simulink model "sampleModel653"  (R2023a)
settings: Solver=VariableStepAuto  StartTime=0.0  StopTime=10.0  RelTol=1e-3
undefined symbols (not defined in the file): DiscIntNeverNeededParam, magnitude, Newton, Raphson
libraries: simulink x238, slpidlib x68
(part 5 of 11)

== system sampleModel653/cfblk133/cfblk4 ==
  cfblk1 : Inport
  cfblk10 : Gain  Gain=[-367085612.698275]
  cfblk11 : Delay  SampleTime=1
  cfblk3 : DiscreteTransferFcn  SampleTime=1
  cfblk4 : Delay  DelayLengthSource=Input port  SampleTime=1
      settings: InputPortMap=u0,p1
  cfblk5 : simulink/Discrete/Transfer Fcn First Order  PoleZ=0.95  ICPrevOutput=0.0  DoSatur=off
  cfblk6 : Polyval  Coefs=[ +2.081618890e-019, -1.441693666e-014, +4.719686976e-010, -8.536869453e-006, +1.621573104e-001, -8.087801117e+001 ]
  cfblk7 : Product  Inputs=*
  cfblk8 : ComplexToMagnitudeAngle
  cfblk9 : Signum
  cfblk2 : Outport
  wires:
  cfblk7/1 -> cfblk5/1
  cfblk8/1 -> cfblk4/1
  cfblk9/1 -> cfblk10/1
  cfblk1/1 -> cfblk4/2
  cfblk10/1 -> cfblk2/1
  cfblk4/1 -> cfblk6/1
  cfblk3/1 -> cfblk8/1
  cfblk6/1 -> cfblk7/1
  cfblk5/1 -> cfblk9/1
  cfblk8/2 -> cfblk11/1
  cfblk11/1 -> cfblk3/1

== system sampleModel653/cfblk133/cfblk5 ==
  cfblk1 : Inport
  cfblk10 : Inport  Port=2
  cfblk11 : Inport  Port=3
  cfblk12 : Inport  Port=4
  cfblk13 : Inport  Port=5
  cfblk3 : simulink/Discrete/Transfer Fcn Real Zero  ZeroZ=0.75  ICPrevInput=0.0  DoSatur=off
  cfblk4 : MinMax  Function=max  Inputs=3
  cfblk5 : MinMax  Inputs=3
  cfblk6 : Sum  Inputs=+
  cfblk7 : Sqrt
  cfblk8 : Signum
  cfblk9 : Constant  Value=[860922626.911465]  SampleTime=1
  cfblk2 : Outport
  wires:
  cfblk5/1 -> cfblk8/1
  cfblk6/1 -> cfblk3/1
  cfblk11/1 -> cfblk2/1
  cfblk13/1 -> cfblk4/1
  cfblk9/1 -> cfblk7/1
  cfblk1/1 -> cfblk5/1
  cfblk8/1 -> cfblk4/2
  cfblk7/1 -> cfblk6/1
  cfblk3/1 -> cfblk4/3
  cfblk10/1 -> cfblk5/2
  cfblk12/1 -> cfblk5/3

== system sampleModel653/cfblk134/cfblk7 ==
  cfblk1 : Inport
  cfblk9 : Inport  Port=2
  cfblk10 : Inport  Port=3
  cfblk11 : Inport  Port=4
  cfblk12 : Inport  Port=5
  cfblk14 : Delay  SampleTime=1
  cfblk15 : Delay  SampleTime=1
  cfblk3 : DiscreteFilter  SampleTime=1
  cfblk4 : Sqrt  Operator=rSqrt  AlgorithmType=Newton-Raphson
  cfblk5 : Product  Inputs=**
  cfblk6 : Abs  SaturateOnIntegerOverflow=off
  cfblk7 : Trigonometry
  cfblk8 : Assignment  DiagnosticForDimensions=Warning  IndexOptions=Index vector (dialog)  Indices=1  OutputSizes=1
  cfblk2 : Outport
  cfblk13 : Outport  Port=2
  wires:
  cfblk1/1 -> cfblk2/1
  cfblk3/1 -> cfblk8/1
  cfblk10/1 -> cfblk3/1
  cfblk12/1 -> cfblk5/1
  cfblk4/1 -> cfblk5/2
  cfblk9/1 -> cfblk8/2
  cfblk6/1 -> cfblk7/1
  cfblk8/1 -> cfblk13/1
  cfblk5/1 -> cfblk14/1
  cfblk14/1 -> cfblk4/1
  cfblk7/1 -> cfblk15/1
  cfblk15/1 -> cfblk6/1

== system sampleModel653/cfblk134/cfblk8 ==
  cfblk1 : Inport
  cfblk12 : Inport  Port=2
  cfblk10 : Reshape
  cfblk11 : Sum  Inputs=|++
  cfblk13 : Delay  SampleTime=1
  cfblk14 : Delay  SampleTime=1
  cfblk3 : simulink/Discrete/Transfer Fcn First Order  PoleZ=0.95  ICPrevOutput=0.0  DoSatur=off
  cfblk4 : DiscreteTransferFcn  SampleTime=1
  cfblk5 : Delay  SampleTime=1
  cfblk6 : Reshape
  cfblk7 : Assignment  DiagnosticForDimensions=Warning  IndexOptions=Index vector (dialog)  Indices=1  OutputSizes=1
  cfblk8 : DotProduct  OutDataTypeStr=Inherit: Inherit via internal rule
  cfblk9 : Reshape
  cfblk2 : Outport
  wires:
  cfblk6/1 -> cfblk2/1
  cfblk1/1 -> cfblk7/1, cfblk8/2
  cfblk12/1 -> cfblk9/1
  cfblk8/1 -> cfblk6/1, cfblk4/1
  cfblk9/1 -> cfblk11/1
  cfblk4/1 -> cfblk11/2
  cfblk7/1 -> cfblk3/1
  cfblk10/1 -> cfblk5/1
  cfblk3/1 -> cfblk10/1
  cfblk5/1 -> cfblk13/1
  cfblk13/1 -> cfblk7/2
  cfblk11/1 -> cfblk14/1
  cfblk14/1 -> cfblk8/1

== system sampleModel653/cfblk135/cfblk7 ==
  cfblk1 : Inport
  cfblk6 : Inport  Port=2
  cfblk7 : Inport  Port=3
  cfblk3 : DiscreteFir  SampleTime=1
  cfblk4 : Rounding
  cfblk5 : Constant  Value=[-731942970.196732]  SampleTime=1
  cfblk2 : Outport
  wires:
  cfblk1/1 -> cfblk3/1
  cfblk3/1 -> cfblk4/1
  cfblk4/1 -> cfblk2/1

== system sampleModel653/cfblk135/cfblk8 ==
  cfblk1 : Inport
  cfblk11 : Inport  Port=2
  cfblk12 : Inport  Port=3
  cfblk13 : Inport  Port=4
  cfblk14 : Inport  Port=5
  cfblk15 : Inport  Port=6
  cfblk10 : Constant  Value=[-864087526.431845]  SampleTime=1
  cfblk3 : Delay  SampleTime=1
  cfblk4 : slpidlib/PID Controller  Controller=PID  Form=Parallel  TimeDomain=Discrete-time  UseExternalTs=off  SampleTime=1  IntegratorMethod=Forward Euler  FilterMethod=Forward Euler  ControllerParametersSource=internal  P=1  I=1  UseKiTs=off  D=0  N=100  UseFilter=on  TunerSelectOption=Transfer Function Based (PID Tuner App)  InitialConditionSource=internal  InitialConditionForIntegrator=0  InitialConditionForFilter=0  DifferentiatorICPrevScaledInput=0  ExternalReset=none  TrackingMode=off  Kt=1  LimitOutput=off  SatLimitsSource=internal  UpperSaturationLimit=inf  LowerSaturationLimit=-inf  LinearizeAsGain=off  AntiWindupMode=none  Kb=1  LimitIntegrator=off  UpperIntegratorSaturationLimit=inf  LowerIntegratorSaturationLimit=-inf  POutMin=[]  POutMax=[]  IOutMin=[]  IOutMax=[]  DOutMin=[]  DOutMax=[]  NOutMin=[]  NOutMax=[]  SumOutMin=[]  SumOutMax=[]  SaturationOutMin=[]  SaturationOutMax=[]  PParamMin=[]  PParamMax=[]  IParamMin=[]  IParamMax=[]  DParamMin=[]  DParamMax=[]  NParamMin=[]  NParamMax=[]  KbParamMin=[]  KbParamMax=[]  KtParamMin=[]  KtParamMax=[]  KbOutMin=[]  KbOutMax=[]  KtOutMin=[]  KtOutMax=[]  IntegratorOutMin=[]  IntegratorOutMax=[]  FilterOutMin=[]  FilterOutMax=[]  SumI1OutMin=[]  SumI1OutMax=[]  SumI2OutMin=[]  SumI2OutMax=[]  SumI3OutMin=[]  SumI3OutMax=[]  SumI4OutMin=[]  SumI4OutMax=[]  SumDOutMin=[]  SumDOutMax=[]  DifferentiatorOutMin=[]  DifferentiatorOutMax=[]  FilterDiffOutCoefMin=[]  FilterDiffOutCoefMax=[]  ReciprocalOutMin=[]  ReciprocalOutMax=[]  SumDenOutMin=[]  SumDenOutMax=[]  SumNumOutMin=[]  SumNumOutMax=[]  DivideOutMin=[]  DivideOutMax=[]  UdiffTsProdOutMin=[]  UdiffTsProdOutMax=[]  NTsProdOutMin=[]  NTsProdOutMax=[]  UintegralTsProdOutMin=[]  UintegralTsProdOutMax=[]  UngainTsProdOutMin=[]  UngainTsProdOutMax=[]  ClampingZeroOutDataTypeStr=Inherit: Inherit via back propagation  ClampingZeroOutMin=[]  ClampingZeroOutMax=[]  FilterDenConstantOutDataTypeStr=Inherit: Inherit via back propagation  FilterDenConstantOutMin=[]  FilterDenConstantOutMax=[]  PCopyOutDataTypeStr=Inherit: Inherit via back propagation  PCopyOutMin=[]  PCopyOutMax=[]  NCopyOutDataTypeStr=Inherit: Inherit via back propagation  NCopyOutMin=[]  NCopyOutMax=[]  IntegratorContinuousStateAttributes=''  IntegratorStateMustResolveToSignalObject=off  IntegratorRTWStateStorageClass=Auto  FilterContinuousStateAttributes=''  FilterStateMustResolveToSignalObject=off  FilterRTWStateStorageClass=Auto  ParallelPVariant=InternalParameters  IdealPVariant=Disabled  IVariant=InternalParameters  DVariant=InternalParameters  IntegratorVariant=Discrete  SatVariant=Disabled  AWVariant=Passthrough  PCopyVariant=Disabled  TRVariant=Disabled  FdbkBlocksVariant=Forward  IdealPFdbkVariant=Disabled  SatFdbkVariant=Disabled  DerivativeFilterVariant=ForwardEulerFilter  NVariant=InternalParameters  NCopyVariant=Disabled  FilterICVariant=InternalICsFilter  IntegratorICVariant=InternalICs  ExternalResetVariant=Disabled  TRSumVariant=Passthrough  SumFdbkVariant=Disabled  SumVariant=Sum_PID  TsampFilterVariant=InternalTs  TsampNgainVariant=Passthrough  TsampIntegralVariant=Disabled_SignalSpec  ExternalSaturationOutDataTypeStr=Inherit: Same as second input
      settings: LibrarySourceBlock=simulink/Discrete/Discrete PID Controller
  cfblk5 : Delay  DelayLengthSource=Input port  SampleTime=1
      settings: InputPortMap=u0,p1
  cfblk6 : Sin  TimeSource=Use external signal  SampleTime=0
  cfblk7 : Rounding
  cfblk8 : Assignment  DiagnosticForDimensions=Warning  IndexOptions=Index vector (dialog)  Indices=1  OutputSizes=1
  cfblk9 : Abs  SaturateOnIntegerOverflow=off
  cfblk2 : Outport
  wires:
  cfblk13/1 -> cfblk5/1
  cfblk12/1 -> cfblk2/1
  cfblk1/1 -> cfblk8/1
  cfblk15/1 -> cfblk9/1
  cfblk8/1 -> cfblk5/2
  cfblk5/1 -> cfblk4/1
  cfblk14/1 -> cfblk3/1
  cfblk11/1 -> cfblk6/1
  cfblk7/1 -> cfblk8/2
  cfblk10/1 -> cfblk7/1

== system sampleModel653/cfblk135/cfblk9 ==
  cfblk1 : Inport
  cfblk12 : Inport  Port=2
  cfblk13 : Inport  Port=3
  cfblk10 : Constant  Value=[-400571818.856096]  SampleTime=1
  cfblk11 : Constant  Value=[918640982.399753]  SampleTime=1
  cfblk15 : Delay  SampleTime=1
  cfblk3 : PropagationDelay  SampleTime=1
  cfblk4 : DiscreteIntegrator  ICPrevOutput=DiscIntNeverNeededParam  ICPrevScaledInput=DiscIntNeverNeededParam
  cfblk5 : simulink/Discrete/Tapped Delay  vinit=0.0  samptime=-1  NumDelays=1  DelayOrder=Oldest  includeCurrent=off
  cfblk6 : PropagationDelay  SampleTime=1
  cfblk7 : DiscreteStateSpace
  cfblk8 : PermuteDimensions
  cfblk9 : MinMax  Function=max  Inputs=2
  cfblk2 : Outport
  cfblk14 : Outport  Port=2
  wires:
  cfblk6/1 -> cfblk9/1
  cfblk7/1 -> cfblk9/2
  cfblk1/1 -> cfblk3/1
  cfblk5/1 -> cfblk8/1
  cfblk12/1 -> cfblk14/1
  cfblk13/1 -> cfblk5/1
  cfblk10/1 -> cfblk3/2
  cfblk11/1 -> cfblk7/1
  cfblk8/1 -> cfblk2/1
  cfblk3/1 -> cfblk4/1
  cfblk4/1 -> cfblk6/1
  cfblk9/1 -> cfblk15/1
  cfblk15/1 -> cfblk6/2

== system sampleModel653/cfblk136/cfblk7 ==
  cfblk1 : Inport
  cfblk13 : Inport  Port=2
  cfblk14 : Inport  Port=3
  cfblk10 : Reshape
  cfblk11 : Constant  Value=[-826386414.772725]  SampleTime=1
  cfblk12 : Constant  Value=[-383763511.639933]  SampleTime=1
  cfblk15 : Delay  SampleTime=1
  cfblk3 : PropagationDelay  SampleTime=1
  cfblk4 : simulink/Discrete/Tapped Delay  vinit=0.0  samptime=-1  NumDelays=1  DelayOrder=Oldest  includeCurrent=off
  cfblk5 : simulink/Discrete/Transfer Fcn Lead or Lag  PoleZ=0.95  ZeroZ=0.75  ICPrevOutput=0.0  ICPrevInput=0.0  DoSatur=off
  cfblk6 : slpidlib/PID Controller (2DOF)  Controller=PID  Form=Parallel  TimeDomain=Discrete-time  UseExternalTs=off  SampleTime=1  IntegratorMethod=Forward Euler  FilterMethod=Forward Euler  ControllerParametersSource=internal  P=1  I=1  UseKiTs=off  D=0  N=100  UseFilter=on  b=1  c=1  TunerSelectOption=Transfer Function Based (PID Tuner App)  InitialConditionSource=internal  InitialConditionForIntegrator=0  InitialConditionForFilter=0  DifferentiatorICPrevScaledInput=0  ExternalReset=none  TrackingMode=off  Kt=1  LimitOutput=off  SatLimitsSource=internal  UpperSaturationLimit=inf  LowerSaturationLimit=-inf  LinearizeAsGain=off  AntiWindupMode=none  Kb=1  LimitIntegrator=off  UpperIntegratorSaturationLimit=inf  LowerIntegratorSaturationLimit=-inf  POutMin=[]  POutMax=[]  IOutMin=[]  IOutMax=[]  DOutMin=[]  DOutMax=[]  NOutMin=[]  NOutMax=[]  bOutMin=[]  bOutMax=[]  cOutMin=[]  cOutMax=[]  SumOutMin=[]  SumOutMax=[]  SaturationOutMin=[]  SaturationOutMax=[]  PParamMin=[]  PParamMax=[]  IParamMin=[]  IParamMax=[]  DParamMin=[]  DParamMax=[]  NParamMin=[]  NParamMax=[]  bParamMin=[]  bParamMax=[]  cParamMin=[]  cParamMax=[]  KbParamMin=[]  KbParamMax=[]  KtParamMin=[]  KtParamMax=[]  KbOutMin=[]  KbOutMax=[]  KtOutMin=[]  KtOutMax=[]  IntegratorOutMin=[]  IntegratorOutMax=[]  FilterOutMin=[]  FilterOutMax=[]  SumI1OutMin=[]  SumI1OutMax=[]  SumI2OutMin=[]  SumI2OutMax=[]  SumI3OutMin=[]  SumI3OutMax=[]  SumI4OutMin=[]  SumI4OutMax=[]  SumDOutMin=[]  SumDOutMax=[]  Sum1OutMin=[]  Sum1OutMax=[]  Sum2OutMin=[]  Sum2OutMax=[]  Sum3OutMin=[]  Sum3OutMax=[]  DifferentiatorOutMin=[]  DifferentiatorOutMax=[]  FilterDiffOutCoefMin=[]  FilterDiffOutCoefMax=[]  ReciprocalOutMin=[]  ReciprocalOutMax=[]  SumDenOutMin=[]  SumDenOutMax=[]  SumNumOutMin=[]  SumNumOutMax=[]  DivideOutMin=[]  DivideOutMax=[]  UdiffTsProdOutMin=[]  UdiffTsProdOutMax=[]  NTsProdOutMin=[]  NTsProdOutMax=[]  UintegralTsProdOutMin=[]  UintegralTsProdOutMax=[]  UngainTsProdOutMin=[]  UngainTsProdOutMax=[]  ClampingZeroOutDataTypeStr=Inherit: Inherit via back propagation  ClampingZeroOutMin=[]  ClampingZeroOutMax=[]  FilterDenConstantOutDataTypeStr=Inherit: Inherit via back propagation  FilterDenConstantOutMin=[]  FilterDenConstantOutMax=[]  PCopyOutDataTypeStr=Inherit: Inherit via back propagation  PCopyOutMin=[]  PCopyOutMax=[]  NCopyOutDataTypeStr=Inherit: Inherit via back propagation  NCopyOutMin=[]  NCopyOutMax=[]  IntegratorContinuousStateAttributes=''  IntegratorStateMustResolveToSignalObject=off  IntegratorRTWStateStorageClass=Auto  FilterContinuousStateAttributes=''  FilterStateMustResolveToSignalObject=off  FilterRTWStateStorageClass=Auto  ParallelPVariant=InternalParameters  IdealPVariant=Disabled  IVariant=InternalParameters  DVariant=InternalParameters  bVariant=InternalParameters  cVariant=InternalParameters  IntegratorVariant=Discrete  SatVariant=Disabled  AWVariant=Passthrough  PCopyVariant=Disabled  TRVariant=Disabled  FdbkBlocksVariant=Forward  IdealPFdbkVariant=Disabled  SatFdbkVariant=Disabled  DerivativeFilterVariant=ForwardEulerFilter  NVariant=InternalParameters  NCopyVariant=Disabled  FilterICVariant=InternalICsFilter  IntegratorICVariant=InternalICs  ExternalResetVariant=Disabled  TRSumVariant=Passthrough  SumFdbkVariant=Disabled  SumVariant=Sum_PID  TsampFilterVariant=InternalTs  TsampNgainVariant=Passthrough  TsampIntegralVariant=Disabled_SignalSpec  ExternalSaturationOutDataTypeStr=Inherit: Same as second input
      settings: LibrarySourceBlock=simulink/Discrete/Discrete PID Controller (2DOF)
  cfblk7 : Gain  Gain=[-873733267.724937]
  cfblk8 : Product  Inputs=*
  cfblk9 : Sin  TimeSource=Use external signal  SampleTime=0
  cfblk2 : Outport
  wires:
  cfblk10/1 -> cfblk9/1
  cfblk12/1 -> cfblk6/1
  cfblk6/1 -> cfblk8/1
  cfblk5/1 -> cfblk6/2
  cfblk3/1 -> cfblk7/1
  cfblk7/1 -> cfblk4/1
  cfblk11/1 -> cfblk10/1
  cfblk9/1 -> cfblk3/1
  cfblk1/1 -> cfblk3/2
  cfblk14/1 -> cfblk2/1
  cfblk8/1 -> cfblk15/1
  cfblk15/1 -> cfblk5/1

== system sampleModel653/cfblk137/cfblk10 ==
  cfblk1 : Inport
  cfblk12 : Inport  Port=2
  cfblk10 : Sum  Inputs=+
  cfblk11 : Constant  Value=[-260614556.659849]  SampleTime=1
  cfblk14 : Delay  SampleTime=1
  cfblk3 : DiscreteFir  SampleTime=1
  cfblk4 : DiscreteZeroPole  Poles=[0 0.5]  Gain=1
  cfblk5 : DiscreteTransferFcn  SampleTime=1
  cfblk6 : Abs  SaturateOnIntegerOverflow=off
  cfblk7 : Gain  Gain=[176697263.776882]
  cfblk8 : Product
  cfblk9 : Sin  TimeSource=Use external signal  SampleTime=0
  cfblk2 : Outport
  cfblk13 : Outport  Port=2
  wires:
  cfblk1/1 -> cfblk10/1
  cfblk5/1 -> cfblk4/1
  cfblk10/1 -> cfblk13/1
  cfblk4/1 -> cfblk7/1
  cfblk12/1 -> cfblk6/1
  cfblk8/1 -> cfblk5/1
  cfblk6/1 -> cfblk8/1
  cfblk11/1 -> cfblk2/1
  cfblk3/1 -> cfblk9/1
  cfblk9/1 -> cfblk8/2
  cfblk7/1 -> cfblk14/1
  cfblk14/1 -> cfblk3/1

== system sampleModel653/cfblk137/cfblk11 ==
  cfblk1 : Inport
  cfblk8 : Inport  Port=2
  cfblk3 : DiscreteIntegrator  ICPrevOutput=DiscIntNeverNeededParam  ICPrevScaledInput=DiscIntNeverNeededParam
  cfblk4 : PropagationDelay  SampleTime=1
  cfblk5 : DiscreteFir  SampleTime=1
  cfblk6 : Sqrt
  cfblk7 : Constant  Value=[22439859.716240]  SampleTime=1
  cfblk9 : Delay  SampleTime=1
  cfblk2 : Outport
  wires:
  cfblk4/1 -> cfblk5/1
  cfblk1/1 -> cfblk2/1
  cfblk7/1 -> cfblk3/1
  cfblk5/1 -> cfblk6/1
  cfblk8/1 -> cfblk4/1
  cfblk6/1 -> cfblk9/1
  cfblk9/1 -> cfblk4/2

== system sampleModel653/cfblk137/cfblk12 ==
  cfblk1 : Inport
  cfblk6 : Inport  Port=2
  cfblk3 : simulink/Discrete/Tapped Delay  vinit=0.0  samptime=-1  NumDelays=1  DelayOrder=Oldest  includeCurrent=off
  cfblk4 : Gain  Gain=[582632264.998820]
  cfblk5 : Sum  Inputs=|++
  cfblk2 : Outport
  cfblk7 : Outport  Port=2
  wires:
  cfblk1/1 -> cfblk5/1, cfblk7/1
  cfblk6/1 -> cfblk5/2
  cfblk3/1 -> cfblk4/1
  cfblk5/1 -> cfblk3/1
  cfblk4/1 -> cfblk2/1

== system sampleModel653/cfblk137/cfblk9 ==
  cfblk1 : Inport
  cfblk7 : Inport  Port=2
  cfblk8 : Inport  Port=3
  cfblk9 : Inport  Port=4
  cfblk10 : Delay  SampleTime=1
  cfblk3 : simulink/Math Operations/MinMax Running Resettable  Function=min  vinit=0.0
  cfblk4 : Squeeze
  cfblk5 : Rounding
  cfblk6 : Product
  cfblk2 : Outport
  wires:
  cfblk6/1 -> cfblk5/1
  cfblk1/1 -> cfblk2/1
  cfblk8/1 -> cfblk3/2
  cfblk5/1 -> cfblk4/1
  cfblk9/1 -> cfblk6/1
  cfblk3/1 -> cfblk6/2
  cfblk4/1 -> cfblk10/1
  cfblk10/1 -> cfblk3/1

== system sampleModel653/cfblk138/cfblk18 ==
  cfblk1 : Inport
  cfblk7 : Inport  Port=2
  Action Port : ActionPort  ActionPortLabel=if(u1 >= 0)
  cfblk3 : Delay  ShowEnablePort=on
      settings: InputPortMap=u0,e6
  cfblk4 : Delay
  cfblk5 : ComplexToRealImag
  cfblk6 : Constant  Value=[554626067.921114]  SampleTime=1
  cfblk2 : Outport
  cfblk8 : Outport  Port=2
  cfblk9 : Outport  Port=3
  wires:
  cfblk7/1 -> cfblk5/1
  cfblk3/1 -> cfblk9/1
  cfblk1/1 -> cfblk8/1
  cfblk6/1 -> cfblk4/1
  cfblk4/1 -> cfblk3/1
  cfblk5/1 -> cfblk3/2
  cfblk5/2 -> cfblk2/1

== system sampleModel653/cfblk138/cfblk19 ==
  cfblk1 : Inport
  cfblk12 : Inport  Port=2
  Action Port : ActionPort  ActionPortLabel=else
  cfblk10 : Constant  Value=[-552232899.805833]  SampleTime=1
  cfblk11 : Constant  Value=[401594460.340258]  SampleTime=1
  cfblk3 : DiscreteFilter
  cfblk4 : Sum  Inputs=|++
  cfblk5 : PermuteDimensions
  cfblk6 : Gain  Gain=[-25396431.824960]
  cfblk7 : Sum  Inputs=|++
  cfblk8 : Bias  Bias=[255966605.717240]  SaturateOnIntegerOverflow=off
  cfblk9 : Constant  Value=[505045263.346821]  SampleTime=1
  cfblk2 : Outport
  cfblk13 : Outport  Port=2
  wires:
  cfblk4/1 -> cfblk13/1
  cfblk9/1 -> cfblk3/1
  cfblk6/1 -> cfblk2/1
  cfblk3/1 -> cfblk6/1
  cfblk11/1 -> cfblk4/1
  cfblk5/1 -> cfblk4/2
  cfblk8/1 -> cfblk7/1
  cfblk10/1 -> cfblk7/2
  cfblk7/1 -> cfblk5/1
  cfblk1/1 -> cfblk8/1

== system sampleModel653/cfblk138/cfblk20 ==
  cfblk1 : Inport
  cfblk13 : Inport  Port=2
  Action Port : ActionPort  ActionPortLabel=if(u1 >= 0)
  cfblk10 : UnaryMinus
  cfblk11 : DotProduct  OutDataTypeStr=Inherit: Inherit via internal rule
  cfblk12 : Product
  cfblk15 : Delay
  cfblk3 : UnitDelay  SampleTime=-1  HasFrameUpgradeWarning=on
  cfblk4 : Delay  ShowEnablePort=on
      settings: InputPortMap=u0,e6
  cfblk5 : UnitDelay  SampleTime=-1  HasFrameUpgradeWarning=on
  cfblk6 : simulink/Discrete/Difference  ICPrevInput=0.0  OutMin=[]  OutMax=[]  OutDataTypeStr=Inherit: Inherit via back propagation  OutDataType=fixdt(1, 16)  OutScaling=2^-10  DoSatur=off
  cfblk7 : Signum
  cfblk8 : Gain  Gain=[-787983042.580818]
  cfblk9 : Abs  SaturateOnIntegerOverflow=off
  cfblk2 : Outport
  cfblk14 : Outport  Port=2
  wires:
  cfblk10/1 -> cfblk4/1
  cfblk4/1 -> cfblk9/1
  cfblk12/1 -> cfblk11/1, cfblk14/1
  cfblk5/1 -> cfblk11/2
  cfblk6/1 -> cfblk4/2
  cfblk1/1 -> cfblk7/1
  cfblk7/1 -> cfblk12/1, cfblk3/1
  cfblk3/1 -> cfblk10/1, cfblk2/1
  cfblk13/1 -> cfblk5/1
  cfblk9/1 -> cfblk8/1
  cfblk11/1 -> cfblk6/1
  cfblk8/1 -> cfblk15/1
  cfblk15/1 -> cfblk12/2

== system sampleModel653/cfblk138/cfblk21 ==
  cfblk1 : Inport
  cfblk11 : Inport  Port=2
  cfblk12 : Inport  Port=3
  Action Port : ActionPort  ActionPortLabel=else
  cfblk10 : Constant  Value=[-603225244.196797]  SampleTime=1
  cfblk3 : slpidlib/PID Controller (2DOF)  Controller=PID  Form=Parallel  TimeDomain=Discrete-time  UseExternalTs=off  SampleTime=-1  IntegratorMethod=Forward Euler  FilterMethod=Forward Euler  ControllerParametersSource=internal  P=1  I=1  UseKiTs=off  D=0  N=100  UseFilter=on  b=1  c=1  TunerSelectOption=Transfer Function Based (PID Tuner App)  InitialConditionSource=internal  InitialConditionForIntegrator=0  InitialConditionForFilter=0  DifferentiatorICPrevScaledInput=0  ExternalReset=none  TrackingMode=off  Kt=1  LimitOutput=off  SatLimitsSource=internal  UpperSaturationLimit=inf  LowerSaturationLimit=-inf  LinearizeAsGain=off  AntiWindupMode=none  Kb=1  LimitIntegrator=off  UpperIntegratorSaturationLimit=inf  LowerIntegratorSaturationLimit=-inf  POutMin=[]  POutMax=[]  IOutMin=[]  IOutMax=[]  DOutMin=[]  DOutMax=[]  NOutMin=[]  NOutMax=[]  bOutMin=[]  bOutMax=[]  cOutMin=[]  cOutMax=[]  SumOutMin=[]  SumOutMax=[]  SaturationOutMin=[]  SaturationOutMax=[]  PParamMin=[]  PParamMax=[]  IParamMin=[]  IParamMax=[]  DParamMin=[]  DParamMax=[]  NParamMin=[]  NParamMax=[]  bParamMin=[]  bParamMax=[]  cParamMin=[]  cParamMax=[]  KbParamMin=[]  KbParamMax=[]  KtParamMin=[]  KtParamMax=[]  KbOutMin=[]  KbOutMax=[]  KtOutMin=[]  KtOutMax=[]  IntegratorOutMin=[]  IntegratorOutMax=[]  FilterOutMin=[]  FilterOutMax=[]  SumI1OutMin=[]  SumI1OutMax=[]  SumI2OutMin=[]  SumI2OutMax=[]  SumI3OutMin=[]  SumI3OutMax=[]  SumI4OutMin=[]  SumI4OutMax=[]  SumDOutMin=[]  SumDOutMax=[]  Sum1OutMin=[]  Sum1OutMax=[]  Sum2OutMin=[]  Sum2OutMax=[]  Sum3OutMin=[]  Sum3OutMax=[]  DifferentiatorOutMin=[]  DifferentiatorOutMax=[]  FilterDiffOutCoefMin=[]  FilterDiffOutCoefMax=[]  ReciprocalOutMin=[]  ReciprocalOutMax=[]  SumDenOutMin=[]  SumDenOutMax=[]  SumNumOutMin=[]  SumNumOutMax=[]  DivideOutMin=[]  DivideOutMax=[]  UdiffTsProdOutMin=[]  UdiffTsProdOutMax=[]  NTsProdOutMin=[]  NTsProdOutMax=[]  UintegralTsProdOutMin=[]  UintegralTsProdOutMax=[]  UngainTsProdOutMin=[]  UngainTsProdOutMax=[]  ClampingZeroOutDataTypeStr=Inherit: Inherit via back propagation  ClampingZeroOutMin=[]  ClampingZeroOutMax=[]  FilterDenConstantOutDataTypeStr=Inherit: Inherit via back propagation  FilterDenConstantOutMin=[]  FilterDenConstantOutMax=[]  PCopyOutDataTypeStr=Inherit: Inherit via back propagation  PCopyOutMin=[]  PCopyOutMax=[]  NCopyOutDataTypeStr=Inherit: Inherit via back propagation  NCopyOutMin=[]  NCopyOutMax=[]  IntegratorContinuousStateAttributes=''  IntegratorStateMustResolveToSignalObject=off  IntegratorRTWStateStorageClass=Auto  FilterContinuousStateAttributes=''  FilterStateMustResolveToSignalObject=off  FilterRTWStateStorageClass=Auto  ParallelPVariant=InternalParameters  IdealPVariant=Disabled  IVariant=InternalParameters  DVariant=InternalParameters  bVariant=InternalParameters  cVariant=InternalParameters  IntegratorVariant=Discrete  SatVariant=Disabled  AWVariant=Passthrough  PCopyVariant=Disabled  TRVariant=Disabled  FdbkBlocksVariant=Forward  IdealPFdbkVariant=Disabled  SatFdbkVariant=Disabled  DerivativeFilterVariant=ForwardEulerFilter  NVariant=InternalParameters  NCopyVariant=Disabled  FilterICVariant=InternalICsFilter  IntegratorICVariant=InternalICs  ExternalResetVariant=Disabled  TRSumVariant=Passthrough  SumFdbkVariant=Disabled  SumVariant=Sum_PID  TsampFilterVariant=InternalTs  TsampNgainVariant=Passthrough  TsampIntegralVariant=Disabled_SignalSpec  ExternalSaturationOutDataTypeStr=Inherit: Same as second input
      settings: LibrarySourceBlock=simulink/Discrete/Discrete PID Controller (2DOF)
  cfblk4 : Sum  Inputs=+
  cfblk5 : Squeeze
  cfblk6 : Gain  Gain=[-505455204.501225]
  cfblk7 : Sin  TimeSource=Use external signal  SampleTime=0
  cfblk8 : Sqrt  Operator=rSqrt  AlgorithmType=Newton-Raphson
  cfblk9 : Product
  cfblk2 : Outport
  wires:
  cfblk1/1 -> cfblk5/1
  cfblk7/1 -> cfblk6/1
  cfblk4/1 -> cfblk9/1
  cfblk5/1 -> cfblk2/1
  cfblk11/1 -> cfblk9/2
  cfblk10/1 -> cfblk7/1
  cfblk8/1 -> cfblk3/1
  cfblk12/1 -> cfblk4/1
  cfblk9/1 -> cfblk3/2
  cfblk6/1 -> cfblk8/1

== system sampleModel653/cfblk138/cfblk22 ==
  cfblk1 : Inport
  cfblk7 : Inport  Port=2
  cfblk8 : Inport  Port=3
  Action Port : ActionPort  ActionPortLabel=if(u1 >= 0)
  cfblk3 : Sqrt  Operator=rSqrt  AlgorithmType=Newton-Raphson
  cfblk4 : UnaryMinus
  cfblk5 : Product  Inputs=**
  cfblk6 : Constant  Value=[-429878194.719558]  SampleTime=1
  cfblk2 : Outport
  wires:
  cfblk1/1 -> cfblk3/1
  cfblk4/1 -> cfblk2/1
  cfblk8/1 -> cfblk4/1
  cfblk6/1 -> cfblk5/1
  cfblk7/1 -> cfblk5/2

== system sampleModel653/cfblk138/cfblk23 ==
  cfblk1 : Inport
  cfblk10 : Inport  Port=2
  cfblk11 : Inport  Port=3
  cfblk12 : Inport  Port=4
  cfblk13 : Inport  Port=5
  cfblk14 : Inport  Port=6
  Action Port : ActionPort  ActionPortLabel=else
  cfblk3 : slpidlib/PID Controller  Controller=PID  Form=Parallel  TimeDomain=Discrete-time  UseExternalTs=off  SampleTime=-1  IntegratorMethod=Forward Euler  FilterMethod=Forward Euler  ControllerParametersSource=internal  P=1  I=1  UseKiTs=off  D=0  N=100  UseFilter=on  TunerSelectOption=Transfer Function Based (PID Tuner App)  InitialConditionSource=internal  InitialConditionForIntegrator=0  InitialConditionForFilter=0  DifferentiatorICPrevScaledInput=0  ExternalReset=none  TrackingMode=off  Kt=1  LimitOutput=off  SatLimitsSource=internal  UpperSaturationLimit=inf  LowerSaturationLimit=-inf  LinearizeAsGain=off  AntiWindupMode=none  Kb=1  LimitIntegrator=off  UpperIntegratorSaturationLimit=inf  LowerIntegratorSaturationLimit=-inf  POutMin=[]  POutMax=[]  IOutMin=[]  IOutMax=[]  DOutMin=[]  DOutMax=[]  NOutMin=[]  NOutMax=[]  SumOutMin=[]  SumOutMax=[]  SaturationOutMin=[]  SaturationOutMax=[]  PParamMin=[]  PParamMax=[]  IParamMin=[]  IParamMax=[]  DParamMin=[]  DParamMax=[]  NParamMin=[]  NParamMax=[]  KbParamMin=[]  KbParamMax=[]  KtParamMin=[]  KtParamMax=[]  KbOutMin=[]  KbOutMax=[]  KtOutMin=[]  KtOutMax=[]  IntegratorOutMin=[]  IntegratorOutMax=[]  FilterOutMin=[]  FilterOutMax=[]  SumI1OutMin=[]  SumI1OutMax=[]  SumI2OutMin=[]  SumI2OutMax=[]  SumI3OutMin=[]  SumI3OutMax=[]  SumI4OutMin=[]  SumI4OutMax=[]  SumDOutMin=[]  SumDOutMax=[]  DifferentiatorOutMin=[]  DifferentiatorOutMax=[]  FilterDiffOutCoefMin=[]  FilterDiffOutCoefMax=[]  ReciprocalOutMin=[]  ReciprocalOutMax=[]  SumDenOutMin=[]  SumDenOutMax=[]  SumNumOutMin=[]  SumNumOutMax=[]  DivideOutMin=[]  DivideOutMax=[]  UdiffTsProdOutMin=[]  UdiffTsProdOutMax=[]  NTsProdOutMin=[]  NTsProdOutMax=[]  UintegralTsProdOutMin=[]  UintegralTsProdOutMax=[]  UngainTsProdOutMin=[]  UngainTsProdOutMax=[]  ClampingZeroOutDataTypeStr=Inherit: Inherit via back propagation  ClampingZeroOutMin=[]  ClampingZeroOutMax=[]  FilterDenConstantOutDataTypeStr=Inherit: Inherit via back propagation  FilterDenConstantOutMin=[]  FilterDenConstantOutMax=[]  PCopyOutDataTypeStr=Inherit: Inherit via back propagation  PCopyOutMin=[]  PCopyOutMax=[]  NCopyOutDataTypeStr=Inherit: Inherit via back propagation  NCopyOutMin=[]  NCopyOutMax=[]  IntegratorContinuousStateAttributes=''  IntegratorStateMustResolveToSignalObject=off  IntegratorRTWStateStorageClass=Auto  FilterContinuousStateAttributes=''  FilterStateMustResolveToSignalObject=off  FilterRTWStateStorageClass=Auto  ParallelPVariant=InternalParameters  IdealPVariant=Disabled  IVariant=InternalParameters  DVariant=InternalParameters  IntegratorVariant=Discrete  SatVariant=Disabled  AWVariant=Passthrough  PCopyVariant=Disabled  TRVariant=Disabled  FdbkBlocksVariant=Forward  IdealPFdbkVariant=Disabled  SatFdbkVariant=Disabled  DerivativeFilterVariant=ForwardEulerFilter  NVariant=InternalParameters  NCopyVariant=Disabled  FilterICVariant=InternalICsFilter  IntegratorICVariant=InternalICs  ExternalResetVariant=Disabled  TRSumVariant=Passthrough  SumFdbkVariant=Disabled  SumVariant=Sum_PID  TsampFilterVariant=InternalTs  TsampNgainVariant=Passthrough  TsampIntegralVariant=Disabled_SignalSpec  ExternalSaturationOutDataTypeStr=Inherit: Same as second input
      settings: LibrarySourceBlock=simulink/Discrete/Discrete PID Controller
  cfblk4 : UnitDelay  SampleTime=-1  HasFrameUpgradeWarning=on
  cfblk5 : UnitDelay  SampleTime=-1  HasFrameUpgradeWarning=on
  cfblk6 : DiscreteZeroPole  Poles=[0 0.5]  Gain=1  SampleTime=-1
  cfblk7 : DiscreteFilter
  cfblk8 : ComplexToMagnitudeAngle
  cfblk9 : Constant  Value=[-513045735.759575]  SampleTime=1
  cfblk2 : Outport
  cfblk15 : Outport  Port=2
  cfblk16 : Outport  Port=3
  cfblk17 : Outport  Port=4
  wires:
  cfblk9/1 -> cfblk7/1
  cfblk5/1 -> cfblk17/1
  cfblk12/1 -> cfblk3/1
  cfblk7/1 -> cfblk15/1
  cfblk8/1 -> cfblk16/1
  cfblk14/1 -> cfblk6/1
  cfblk13/1 -> cfblk8/1
  cfblk8/2 -> cfblk4/1
  cfblk4/1 -> cfblk5/1
  cfblk6/1 -> cfblk2/1

== system sampleModel653/cfblk138/cfblk8 ==
  cfblk1 : Inport
  cfblk7 : Inport  Port=2
  cfblk3 : Sum  Inputs=+
  cfblk4 : Abs  SaturateOnIntegerOverflow=off
  cfblk5 : Constant  Value=[-577316308.345091]  SampleTime=1
  cfblk6 : Constant  Value=[-337681300.879887]  SampleTime=1
  cfblk2 : Outport
  cfblk8 : Outport  Port=2
  wires:
  cfblk4/1 -> cfblk2/1
  cfblk7/1 -> cfblk8/1
  cfblk1/1 -> cfblk3/1
  cfblk6/1 -> cfblk4/1

== system sampleModel653/cfblk138/cfblk9 ==
  cfblk1 : Inport
  cfblk12 : Inport  Port=2
  cfblk10 : Constant  Value=[292063134.196269]  SampleTime=1
  cfblk11 : Constant  Value=[977331513.676573]  SampleTime=1
  cfblk3 : DiscreteTransferFcn  SampleTime=1
  cfblk4 : Delay  DelayLengthSource=Input port  SampleTime=1
      settings: InputPortMap=u0,p1
  cfblk5 : Gain  Gain=[-397270948.820147]
  cfblk6 : ComplexToRealImag
  cfblk7 : ComplexToMagnitudeAngle
  cfblk8 : Signum
  cfblk9 : Bias  Bias=[-964054982.827506]  SaturateOnIntegerOverflow=off
  cfblk2 : Outport
  cfblk13 : Outport  Port=2
  cfblk14 : Outport  Port=3
  wires:
  cfblk3/1 -> cfblk5/1
  cfblk6/1 -> cfblk2/1
  cfblk9/1 -> cfblk6/1
  cfblk12/1 -> cfblk8/1
  cfblk1/1 -> cfblk13/1
  cfblk4/1 -> cfblk7/1
  cfblk6/2 -> cfblk14/1
  cfblk8/1 -> cfblk3/1
  cfblk5/1 -> cfblk4/1
  cfblk11/1 -> cfblk4/2
  cfblk7/1 -> cfblk9/1

== system sampleModel653/cfblk139/cfblk10 ==
  cfblk1 : Inport
  cfblk7 : Inport  Port=2
  cfblk10 : Delay  SampleTime=1
  cfblk3 : simulink/Discrete/Difference  ICPrevInput=0.0  OutMin=[]  OutMax=[]  OutDataTypeStr=Inherit: Inherit via back propagation  OutDataType=fixdt(1, 16)  OutScaling=2^-10  DoSatur=off
  cfblk4 : Delay  DelayLengthSource=Input port  SampleTime=1
      settings: InputPortMap=u0,p1
  cfblk5 : Sqrt
  cfblk6 : Trigonometry
  cfblk2 : Outport
  cfblk8 : Outport  Port=2
  cfblk9 : Outport  Port=3
  wires:
  cfblk5/1 -> cfblk8/1
  cfblk6/1 -> cfblk3/1
  cfblk3/1 -> cfblk2/1, cfblk10/1
  cfblk7/1 -> cfblk9/1
  cfblk1/1 -> cfblk4/1
  cfblk4/1 -> cfblk6/1, cfblk5/1
  cfblk10/1 -> cfblk4/2

== system sampleModel653/cfblk139/cfblk11 ==
  cfblk1 : Inport
  cfblk12 : Inport  Port=2
  cfblk13 : Inport  Port=3
  cfblk14 : Inport  Port=4
  cfblk15 : Inport  Port=5
  cfblk16 : Inport  Port=6
  cfblk10 : Constant  Value=[-994427606.481637]  SampleTime=1
  cfblk11 : Constant  Value=[-26386766.859515]  SampleTime=1
  cfblk17 : Delay  SampleTime=1
  cfblk3 : PropagationDelay  SampleTime=1
  cfblk4 : DiscreteStateSpace
  cfblk5 : DiscreteTransferFcn  SampleTime=1
  cfblk6 : Delay  ShowEnablePort=on  SampleTime=1
      settings: InputPortMap=u0,e6
  cfblk7 : ComplexToRealImag
  cfblk8 : Product  Inputs=*
  cfblk9 : Math  Operator=pow
  cfblk2 : Outport
  wires:
  cfblk10/1 -> cfblk6/1
  cfblk16/1 -> cfblk3/1
  cfblk6/1 -> cfblk9/1
  cfblk12/1 -> cfblk9/2
  cfblk3/1 -> cfblk2/1
  cfblk7/1 -> cfblk3/2
  cfblk11/1 -> cfblk8/1
  cfblk5/1 -> cfblk6/2
  cfblk14/1 -> cfblk7/1
  cfblk1/1 -> cfblk4/1
  cfblk9/1 -> cfblk17/1
  cfblk17/1 -> cfblk5/1

== system sampleModel653/cfblk139/cfblk12 ==
  cfblk1 : Inport
  cfblk10 : Inport  Port=2
  cfblk14 : Delay  SampleTime=1
  cfblk3 : DiscreteZeroPole  Poles=[0 0.5]  Gain=1
  cfblk4 : slpidlib/PID Controller (2DOF)  Controller=PID  Form=Parallel  TimeDomain=Discrete-time  UseExternalTs=off  SampleTime=1  IntegratorMethod=Forward Euler  FilterMethod=Forward Euler  ControllerParametersSource=internal  P=1  I=1  UseKiTs=off  D=0  N=100  UseFilter=on  b=1  c=1  TunerSelectOption=Transfer Function Based (PID Tuner App)  InitialConditionSource=internal  InitialConditionForIntegrator=0  InitialConditionForFilter=0  DifferentiatorICPrevScaledInput=0  ExternalReset=none  TrackingMode=off  Kt=1  LimitOutput=off  SatLimitsSource=internal  UpperSaturationLimit=inf  LowerSaturationLimit=-inf  LinearizeAsGain=off  AntiWindupMode=none  Kb=1  LimitIntegrator=off  UpperIntegratorSaturationLimit=inf  LowerIntegratorSaturationLimit=-inf  POutMin=[]  POutMax=[]  IOutMin=[]  IOutMax=[]  DOutMin=[]  DOutMax=[]  NOutMin=[]  NOutMax=[]  bOutMin=[]  bOutMax=[]  cOutMin=[]  cOutMax=[]  SumOutMin=[]  SumOutMax=[]  SaturationOutMin=[]  SaturationOutMax=[]  PParamMin=[]  PParamMax=[]  IParamMin=[]  IParamMax=[]  DParamMin=[]  DParamMax=[]  NParamMin=[]  NParamMax=[]  bParamMin=[]  bParamMax=[]  cParamMin=[]  cParamMax=[]  KbParamMin=[]  KbParamMax=[]  KtParamMin=[]  KtParamMax=[]  KbOutMin=[]  KbOutMax=[]  KtOutMin=[]  KtOutMax=[]  IntegratorOutMin=[]  IntegratorOutMax=[]  FilterOutMin=[]  FilterOutMax=[]  SumI1OutMin=[]  SumI1OutMax=[]  SumI2OutMin=[]  SumI2OutMax=[]  SumI3OutMin=[]  SumI3OutMax=[]  SumI4OutMin=[]  SumI4OutMax=[]  SumDOutMin=[]  SumDOutMax=[]  Sum1OutMin=[]  Sum1OutMax=[]  Sum2OutMin=[]  Sum2OutMax=[]  Sum3OutMin=[]  Sum3OutMax=[]  DifferentiatorOutMin=[]  DifferentiatorOutMax=[]  FilterDiffOutCoefMin=[]  FilterDiffOutCoefMax=[]  ReciprocalOutMin=[]  ReciprocalOutMax=[]  SumDenOutMin=[]  SumDenOutMax=[]  SumNumOutMin=[]  SumNumOutMax=[]  DivideOutMin=[]  DivideOutMax=[]  UdiffTsProdOutMin=[]  UdiffTsProdOutMax=[]  NTsProdOutMin=[]  NTsProdOutMax=[]  UintegralTsProdOutMin=[]  UintegralTsProdOutMax=[]  UngainTsProdOutMin=[]  UngainTsProdOutMax=[]  ClampingZeroOutDataTypeStr=Inherit: Inherit via back propagation  ClampingZeroOutMin=[]  ClampingZeroOutMax=[]  FilterDenConstantOutDataTypeStr=Inherit: Inherit via back propagation  FilterDenConstantOutMin=[]  FilterDenConstantOutMax=[]  PCopyOutDataTypeStr=Inherit: Inherit via back propagation  PCopyOutMin=[]  PCopyOutMax=[]  NCopyOutDataTypeStr=Inherit: Inherit via back propagation  NCopyOutMin=[]  NCopyOutMax=[]  IntegratorContinuousStateAttributes=''  IntegratorStateMustResolveToSignalObject=off  IntegratorRTWStateStorageClass=Auto  FilterContinuousStateAttributes=''  FilterStateMustResolveToSignalObject=off  FilterRTWStateStorageClass=Auto  ParallelPVariant=InternalParameters  IdealPVariant=Disabled  IVariant=InternalParameters  DVariant=InternalParameters  bVariant=InternalParameters  cVariant=InternalParameters  IntegratorVariant=Discrete  SatVariant=Disabled  AWVariant=Passthrough  PCopyVariant=Disabled  TRVariant=Disabled  FdbkBlocksVariant=Forward  IdealPFdbkVariant=Disabled  SatFdbkVariant=Disabled  DerivativeFilterVariant=ForwardEulerFilter  NVariant=InternalParameters  NCopyVariant=Disabled  FilterICVariant=InternalICsFilter  IntegratorICVariant=InternalICs  ExternalResetVariant=Disabled  TRSumVariant=Passthrough  SumFdbkVariant=Disabled  SumVariant=Sum_PID  TsampFilterVariant=InternalTs  TsampNgainVariant=Passthrough  TsampIntegralVariant=Disabled_SignalSpec  ExternalSaturationOutDataTypeStr=Inherit: Same as second input
      settings: LibrarySourceBlock=simulink/Discrete/Discrete PID Controller (2DOF)
  cfblk5 : Delay  ShowEnablePort=on  SampleTime=1
      settings: InputPortMap=u0,e6
  cfblk6 : DotProduct  OutDataTypeStr=Inherit: Inherit via internal rule
  cfblk7 : Sum  Inputs=|++
  cfblk8 : PermuteDimensions
  cfblk9 : Constant  Value=[609204184.320349]  SampleTime=1
  cfblk2 : Outport
  cfblk11 : Outport  Port=2
  cfblk12 : Outport  Port=3
  cfblk13 : Outport  Port=4
  wires:
  cfblk4/1 -> cfblk13/1
  cfblk8/1 -> cfblk7/1, cfblk7/2
  cfblk3/1 -> cfblk4/1, cfblk8/1
  cfblk9/1 -> cfblk11/1
  cfblk5/1 -> cfblk4/2, cfblk6/1, cfblk2/1
  cfblk1/1 -> cfblk3/1
  cfblk10/1 -> cfblk12/1
  cfblk7/1 -> cfblk5/2, cfblk6/2
  cfblk6/1 -> cfblk14/1
  cfblk14/1 -> cfblk5/1

== system sampleModel653/cfblk139/cfblk13 ==
  cfblk1 : Inport
  cfblk6 : Inport  Port=2
  cfblk7 : Inport  Port=3
  cfblk8 : Inport  Port=4
  cfblk3 : DiscreteFilter  SampleTime=1
  cfblk4 : Product  Inputs=**
  cfblk5 : Product  Inputs=*
  cfblk2 : Outport
  wires:
  cfblk5/1 -> cfblk2/1
  cfblk6/1 -> cfblk4/1
  cfblk8/1 -> cfblk3/1
  cfblk1/1 -> cfblk5/1
  cfblk3/1 -> cfblk4/2

== system sampleModel653/cfblk140/cfblk4 ==
  cfblk1 : Inport
  cfblk11 : Inport  Port=2
  cfblk12 : Inport  Port=3
  cfblk13 : Inport  Port=4
  cfblk10 : simulink/Math Operations/Slider Gain  gain=1  low=0  high=2
  cfblk3 : slpidlib/PID Controller (2DOF)  Controller=PID  Form=Parallel  TimeDomain=Discrete-time  UseExternalTs=off  SampleTime=1  IntegratorMethod=Forward Euler  FilterMethod=Forward Euler  ControllerParametersSource=internal  P=1  I=1  UseKiTs=off  D=0  N=100  UseFilter=on  b=1  c=1  TunerSelectOption=Transfer Function Based (PID Tuner App)  InitialConditionSource=internal  InitialConditionForIntegrator=0  InitialConditionForFilter=0  DifferentiatorICPrevScaledInput=0  ExternalReset=none  TrackingMode=off  Kt=1  LimitOutput=off  SatLimitsSource=internal  UpperSaturationLimit=inf  LowerSaturationLimit=-inf  LinearizeAsGain=off  AntiWindupMode=none  Kb=1  LimitIntegrator=off  UpperIntegratorSaturationLimit=inf  LowerIntegratorSaturationLimit=-inf  POutMin=[]  POutMax=[]  IOutMin=[]  IOutMax=[]  DOutMin=[]  DOutMax=[]  NOutMin=[]  NOutMax=[]  bOutMin=[]  bOutMax=[]  cOutMin=[]  cOutMax=[]  SumOutMin=[]  SumOutMax=[]  SaturationOutMin=[]  SaturationOutMax=[]  PParamMin=[]  PParamMax=[]  IParamMin=[]  IParamMax=[]  DParamMin=[]  DParamMax=[]  NParamMin=[]  NParamMax=[]  bParamMin=[]  bParamMax=[]  cParamMin=[]  cParamMax=[]  KbParamMin=[]  KbParamMax=[]  KtParamMin=[]  KtParamMax=[]  KbOutMin=[]  KbOutMax=[]  KtOutMin=[]  KtOutMax=[]  IntegratorOutMin=[]  IntegratorOutMax=[]  FilterOutMin=[]  FilterOutMax=[]  SumI1OutMin=[]  SumI1OutMax=[]  SumI2OutMin=[]  SumI2OutMax=[]  SumI3OutMin=[]  SumI3OutMax=[]  SumI4OutMin=[]  SumI4OutMax=[]  SumDOutMin=[]  SumDOutMax=[]  Sum1OutMin=[]  Sum1OutMax=[]  Sum2OutMin=[]  Sum2OutMax=[]  Sum3OutMin=[]  Sum3OutMax=[]  DifferentiatorOutMin=[]  DifferentiatorOutMax=[]  FilterDiffOutCoefMin=[]  FilterDiffOutCoefMax=[]  ReciprocalOutMin=[]  ReciprocalOutMax=[]  SumDenOutMin=[]  SumDenOutMax=[]  SumNumOutMin=[]  SumNumOutMax=[]  DivideOutMin=[]  DivideOutMax=[]  UdiffTsProdOutMin=[]  UdiffTsProdOutMax=[]  NTsProdOutMin=[]  NTsProdOutMax=[]  UintegralTsProdOutMin=[]  UintegralTsProdOutMax=[]  UngainTsProdOutMin=[]  UngainTsProdOutMax=[]  ClampingZeroOutDataTypeStr=Inherit: Inherit via back propagation  ClampingZeroOutMin=[]  ClampingZeroOutMax=[]  FilterDenConstantOutDataTypeStr=Inherit: Inherit via back propagation  FilterDenConstantOutMin=[]  FilterDenConstantOutMax=[]  PCopyOutDataTypeStr=Inherit: Inherit via back propagation  PCopyOutMin=[]  PCopyOutMax=[]  NCopyOutDataTypeStr=Inherit: Inherit via back propagation  NCopyOutMin=[]  NCopyOutMax=[]  IntegratorContinuousStateAttributes=''  IntegratorStateMustResolveToSignalObject=off  IntegratorRTWStateStorageClass=Auto  FilterContinuousStateAttributes=''  FilterStateMustResolveToSignalObject=off  FilterRTWStateStorageClass=Auto  ParallelPVariant=InternalParameters  IdealPVariant=Disabled  IVariant=InternalParameters  DVariant=InternalParameters  bVariant=InternalParameters  cVariant=InternalParameters  IntegratorVariant=Discrete  SatVariant=Disabled  AWVariant=Passthrough  PCopyVariant=Disabled  TRVariant=Disabled  FdbkBlocksVariant=Forward  IdealPFdbkVariant=Disabled  SatFdbkVariant=Disabled  DerivativeFilterVariant=ForwardEulerFilter  NVariant=InternalParameters  NCopyVariant=Disabled  FilterICVariant=InternalICsFilter  IntegratorICVariant=InternalICs  ExternalResetVariant=Disabled  TRSumVariant=Passthrough  SumFdbkVariant=Disabled  SumVariant=Sum_PID  TsampFilterVariant=InternalTs  TsampNgainVariant=Passthrough  TsampIntegralVariant=Disabled_SignalSpec  ExternalSaturationOutDataTypeStr=Inherit: Same as second input
      settings: LibrarySourceBlock=simulink/Discrete/Discrete PID Controller (2DOF)
  cfblk4 : simulink/Discrete/Transfer Fcn Real Zero  ZeroZ=0.75  ICPrevInput=0.0  DoSatur=off
  cfblk5 : DiscreteFir  SampleTime=1
  cfblk6 : DiscreteFir  SampleTime=1
  cfblk7 : DiscreteFilter  SampleTime=1
  cfblk8 : DiscreteFir  SampleTime=1
  cfblk9 : Math  Operator=transpose
  cfblk2 : Outport
  cfblk14 : Outport  Port=2
  wires:
  cfblk6/1 -> cfblk14/1
  cfblk4/1 -> cfblk6/1
  cfblk5/1 -> cfblk7/1
  cfblk10/1 -> cfblk5/1
  cfblk1/1 -> cfblk10/1
  cfblk8/1 -> cfblk9/1
  cfblk12/1 -> cfblk4/1
  cfblk9/1 -> cfblk3/1
  cfblk11/1 -> cfblk3/2
  cfblk7/1 -> cfblk8/1
  cfblk13/1 -> cfblk2/1

== system sampleModel653/cfblk140/cfblk5 ==
  cfblk1 : Inport
  cfblk7 : Inport  Port=2
  cfblk8 : Inport  Port=3
  cfblk3 : PropagationDelay  SampleTime=1
  cfblk4 : Delay  DelayLengthSource=Input port  SampleTime=1
      settings: InputPortMap=u0,p1
  cfblk5 : Signum
  cfblk6 : UnaryMinus
  cfblk2 : Outport
  wires:
  cfblk5/1 -> cfblk4/1
  cfblk6/1 -> cfblk5/1
  cfblk7/1 -> cfblk4/2
  cfblk1/1 -> cfblk6/1
  cfblk4/1 -> cfblk3/1
  cfblk8/1 -> cfblk3/2
  cfblk3/1 -> cfblk2/1

== system sampleModel653/cfblk140/cfblk6 ==
  cfblk1 : Inport
  cfblk4 : Inport  Port=2
  cfblk5 : Inport  Port=3
  cfblk6 : Inport  Port=4
  cfblk7 : Inport  Port=5
  cfblk3 : slpidlib/PID Controller (2DOF)  Controller=PID  Form=Parallel  TimeDomain=Discrete-time  UseExternalTs=off  SampleTime=1  IntegratorMethod=Forward Euler  FilterMethod=Forward Euler  ControllerParametersSource=internal  P=1  I=1  UseKiTs=off  D=0  N=100  UseFilter=on  b=1  c=1  TunerSelectOption=Transfer Function Based (PID Tuner App)  InitialConditionSource=internal  InitialConditionForIntegrator=0  InitialConditionForFilter=0  DifferentiatorICPrevScaledInput=0  ExternalReset=none  TrackingMode=off  Kt=1  LimitOutput=off  SatLimitsSource=internal  UpperSaturationLimit=inf  LowerSaturationLimit=-inf  LinearizeAsGain=off  AntiWindupMode=none  Kb=1  LimitIntegrator=off  UpperIntegratorSaturationLimit=inf  LowerIntegratorSaturationLimit=-inf  POutMin=[]  POutMax=[]  IOutMin=[]  IOutMax=[]  DOutMin=[]  DOutMax=[]  NOutMin=[]  NOutMax=[]  bOutMin=[]  bOutMax=[]  cOutMin=[]  cOutMax=[]  SumOutMin=[]  SumOutMax=[]  SaturationOutMin=[]  SaturationOutMax=[]  PParamMin=[]  PParamMax=[]  IParamMin=[]  IParamMax=[]  DParamMin=[]  DParamMax=[]  NParamMin=[]  NParamMax=[]  bParamMin=[]  bParamMax=[]  cParamMin=[]  cParamMax=[]  KbParamMin=[]  KbParamMax=[]  KtParamMin=[]  KtParamMax=[]  KbOutMin=[]  KbOutMax=[]  KtOutMin=[]  KtOutMax=[]  IntegratorOutMin=[]  IntegratorOutMax=[]  FilterOutMin=[]  FilterOutMax=[]  SumI1OutMin=[]  SumI1OutMax=[]  SumI2OutMin=[]  SumI2OutMax=[]  SumI3OutMin=[]  SumI3OutMax=[]  SumI4OutMin=[]  SumI4OutMax=[]  SumDOutMin=[]  SumDOutMax=[]  Sum1OutMin=[]  Sum1OutMax=[]  Sum2OutMin=[]  Sum2OutMax=[]  Sum3OutMin=[]  Sum3OutMax=[]  DifferentiatorOutMin=[]  DifferentiatorOutMax=[]  FilterDiffOutCoefMin=[]  FilterDiffOutCoefMax=[]  ReciprocalOutMin=[]  ReciprocalOutMax=[]  SumDenOutMin=[]  SumDenOutMax=[]  SumNumOutMin=[]  SumNumOutMax=[]  DivideOutMin=[]  DivideOutMax=[]  UdiffTsProdOutMin=[]  UdiffTsProdOutMax=[]  NTsProdOutMin=[]  NTsProdOutMax=[]  UintegralTsProdOutMin=[]  UintegralTsProdOutMax=[]  UngainTsProdOutMin=[]  UngainTsProdOutMax=[]  ClampingZeroOutDataTypeStr=Inherit: Inherit via back propagation  ClampingZeroOutMin=[]  ClampingZeroOutMax=[]  FilterDenConstantOutDataTypeStr=Inherit: Inherit via back propagation  FilterDenConstantOutMin=[]  FilterDenConstantOutMax=[]  PCopyOutDataTypeStr=Inherit: Inherit via back propagation  PCopyOutMin=[]  PCopyOutMax=[]  NCopyOutDataTypeStr=Inherit: Inherit via back propagation  NCopyOutMin=[]  NCopyOutMax=[]  IntegratorContinuousStateAttributes=''  IntegratorStateMustResolveToSignalObject=off  IntegratorRTWStateStorageClass=Auto  FilterContinuousStateAttributes=''  FilterStateMustResolveToSignalObject=off  FilterRTWStateStorageClass=Auto  ParallelPVariant=InternalParameters  IdealPVariant=Disabled  IVariant=InternalParameters  DVariant=InternalParameters  bVariant=InternalParameters  cVariant=InternalParameters  IntegratorVariant=Discrete  SatVariant=Disabled  AWVariant=Passthrough  PCopyVariant=Disabled  TRVariant=Disabled  FdbkBlocksVariant=Forward  IdealPFdbkVariant=Disabled  SatFdbkVariant=Disabled  DerivativeFilterVariant=ForwardEulerFilter  NVariant=InternalParameters  NCopyVariant=Disabled  FilterICVariant=InternalICsFilter  IntegratorICVariant=InternalICs  ExternalResetVariant=Disabled  TRSumVariant=Passthrough  SumFdbkVariant=Disabled  SumVariant=Sum_PID  TsampFilterVariant=InternalTs  TsampNgainVariant=Passthrough  TsampIntegralVariant=Disabled_SignalSpec  ExternalSaturationOutDataTypeStr=Inherit: Same as second input
      settings: LibrarySourceBlock=simulink/Discrete/Discrete PID Controller (2DOF)
  cfblk2 : Outport
  wires:
  cfblk6/1 -> cfblk3/1
  cfblk1/1 -> cfblk3/2
  cfblk7/1 -> cfblk2/1

== system sampleModel653/cfblk142/cfblk10 ==
  cfblk1 : Inport
  cfblk10 : Inport  Port=2
  cfblk3 : simulink/Discrete/Difference  ICPrevInput=0.0  OutMin=[]  OutMax=[]  OutDataTypeStr=Inherit: Inherit via back propagation  OutDataType=fixdt(1, 16)  OutScaling=2^-10  DoSatur=off
  cfblk4 : UnitDelay  HasFrameUpgradeWarning=on
  cfblk5 : Abs  SaturateOnIntegerOverflow=off
  cfblk6 : PermuteDimensions
  cfblk7 : Rounding
  cfblk8 : Constant  Value=[-225872583.397093]  SampleTime=1
  cfblk9 : Constant  Value=[-646446268.863192]  SampleTime=1
  cfblk2 : Outport
  cfblk11 : Outport  Port=2
  wires:
  cfblk1/1 -> cfblk3/1
  cfblk6/1 -> cfblk4/1
  cfblk9/1 -> cfblk6/1
  cfblk4/1 -> cfblk11/1
  cfblk5/1 -> cfblk7/1
  cfblk3/1 -> cfblk2/1
  cfblk10/1 -> cfblk5/1

== system sampleModel653/cfblk142/cfblk11 ==
  cfblk1 : Inport
  cfblk11 : Inport  Port=2
  cfblk12 : Inport  Port=3
  cfblk13 : Inport  Port=4
  cfblk10 : Product  Inputs=**
  cfblk3 : Delay  DelayLengthSource=Input port  SampleTime=1
      settings: InputPortMap=u0,p1
  cfblk4 : slpidlib/PID Controller (2DOF)  Controller=PID  Form=Parallel  TimeDomain=Discrete-time  UseExternalTs=off  SampleTime=1  IntegratorMethod=Forward Euler  FilterMethod=Forward Euler  ControllerParametersSource=internal  P=1  I=1  UseKiTs=off  D=0  N=100  UseFilter=on  b=1  c=1  TunerSelectOption=Transfer Function Based (PID Tuner App)  InitialConditionSource=internal  InitialConditionForIntegrator=0  InitialConditionForFilter=0  DifferentiatorICPrevScaledInput=0  ExternalReset=none  TrackingMode=off  Kt=1  LimitOutput=off  SatLimitsSource=internal  UpperSaturationLimit=inf  LowerSaturationLimit=-inf  LinearizeAsGain=off  AntiWindupMode=none  Kb=1  LimitIntegrator=off  UpperIntegratorSaturationLimit=inf  LowerIntegratorSaturationLimit=-inf  POutMin=[]  POutMax=[]  IOutMin=[]  IOutMax=[]  DOutMin=[]  DOutMax=[]  NOutMin=[]  NOutMax=[]  bOutMin=[]  bOutMax=[]  cOutMin=[]  cOutMax=[]  SumOutMin=[]  SumOutMax=[]  SaturationOutMin=[]  SaturationOutMax=[]  PParamMin=[]  PParamMax=[]  IParamMin=[]  IParamMax=[]  DParamMin=[]  DParamMax=[]  NParamMin=[]  NParamMax=[]  bParamMin=[]  bParamMax=[]  cParamMin=[]  cParamMax=[]  KbParamMin=[]  KbParamMax=[]  KtParamMin=[]  KtParamMax=[]  KbOutMin=[]  KbOutMax=[]  KtOutMin=[]  KtOutMax=[]  IntegratorOutMin=[]  IntegratorOutMax=[]  FilterOutMin=[]  FilterOutMax=[]  SumI1OutMin=[]  SumI1OutMax=[]  SumI2OutMin=[]  SumI2OutMax=[]  SumI3OutMin=[]  SumI3OutMax=[]  SumI4OutMin=[]  SumI4OutMax=[]  SumDOutMin=[]  SumDOutMax=[]  Sum1OutMin=[]  Sum1OutMax=[]  Sum2OutMin=[]  Sum2OutMax=[]  Sum3OutMin=[]  Sum3OutMax=[]  DifferentiatorOutMin=[]  DifferentiatorOutMax=[]  FilterDiffOutCoefMin=[]  FilterDiffOutCoefMax=[]  ReciprocalOutMin=[]  ReciprocalOutMax=[]  SumDenOutMin=[]  SumDenOutMax=[]  SumNumOutMin=[]  SumNumOutMax=[]  DivideOutMin=[]  DivideOutMax=[]  UdiffTsProdOutMin=[]  UdiffTsProdOutMax=[]  NTsProdOutMin=[]  NTsProdOutMax=[]  UintegralTsProdOutMin=[]  UintegralTsProdOutMax=[]  UngainTsProdOutMin=[]  UngainTsProdOutMax=[]  ClampingZeroOutDataTypeStr=Inherit: Inherit via back propagation  ClampingZeroOutMin=[]  ClampingZeroOutMax=[]  FilterDenConstantOutDataTypeStr=Inherit: Inherit via back propagation  FilterDenConstantOutMin=[]  FilterDenConstantOutMax=[]  PCopyOutDataTypeStr=Inherit: Inherit via back propagation  PCopyOutMin=[]  PCopyOutMax=[]  NCopyOutDataTypeStr=Inherit: Inherit via back propagation  NCopyOutMin=[]  NCopyOutMax=[]  IntegratorContinuousStateAttributes=''  IntegratorStateMustResolveToSignalObject=off  IntegratorRTWStateStorageClass=Auto  FilterContinuousStateAttributes=''  FilterStateMustResolveToSignalObject=off  FilterRTWStateStorageClass=Auto  ParallelPVariant=InternalParameters  IdealPVariant=Disabled  IVariant=InternalParameters  DVariant=InternalParameters  bVariant=InternalParameters  cVariant=InternalParameters  IntegratorVariant=Discrete  SatVariant=Disabled  AWVariant=Passthrough  PCopyVariant=Disabled  TRVariant=Disabled  FdbkBlocksVariant=Forward  IdealPFdbkVariant=Disabled  SatFdbkVariant=Disabled  DerivativeFilterVariant=ForwardEulerFilter  NVariant=InternalParameters  NCopyVariant=Disabled  FilterICVariant=InternalICsFilter  IntegratorICVariant=InternalICs  ExternalResetVariant=Disabled  TRSumVariant=Passthrough  SumFdbkVariant=Disabled  SumVariant=Sum_PID  TsampFilterVariant=InternalTs  TsampNgainVariant=Passthrough  TsampIntegralVariant=Disabled_SignalSpec  ExternalSaturationOutDataTypeStr=Inherit: Same as second input
      settings: LibrarySourceBlock=simulink/Discrete/Discrete PID Controller (2DOF)
  cfblk5 : UnitDelay  HasFrameUpgradeWarning=on
  cfblk6 : DiscreteIntegrator  ICPrevOutput=DiscIntNeverNeededParam  ICPrevScaledInput=DiscIntNeverNeededParam
  cfblk7 : DiscreteTransferFcn  SampleTime=1
  cfblk8 : Math  Operator=conj
  cfblk9 : UnaryMinus
  cfblk2 : Outport
  wires:
  cfblk7/1 -> cfblk9/1
  cfblk3/1 -> cfblk7/1
  cfblk1/1 -> cfblk8/1
  cfblk11/1 -> cfblk5/1
  cfblk9/1 -> cfblk10/1
  cfblk8/1 -> cfblk4/1
  cfblk13/1 -> cfblk3/1
  cfblk6/1 -> cfblk2/1
  cfblk12/1 -> cfblk4/2
  cfblk5/1 -> cfblk3/2
  cfblk10/1 -> cfblk6/1
  cfblk4/1 -> cfblk10/2
